simulink model "Flowchart5"  (Simulink 6.0)
settings: Solver=FixedStepDiscrete  StartTime=0.0  StopTime=10.0  RelTol=1e-3
settings Model: Creator=scaife  LastModifiedBy=scaife  ExtModeAutoUpdateStatusClock=off

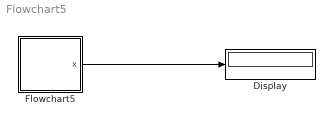
== system Flowchart5 ==
  Display : Display
  Flowchart5 : Stateflow chart
  wires:
  Flowchart5/1(x) -> Display/1

== stateflow chart Flowchart5 ==
  state A [parallel]
    (junction 4) -> (junction 5) : {x++;}
    A -> (junction 4)
    (default) -> (junction 4)
  data: x output int32
